simulink model "add_sine_waves"  (R2021b)
settings: Solver=VariableStepAuto  StartTime=0.0  StopTime=10.0  RelTol=1e-3
settings Model: Creator=emre-  LastModifiedBy=emre-

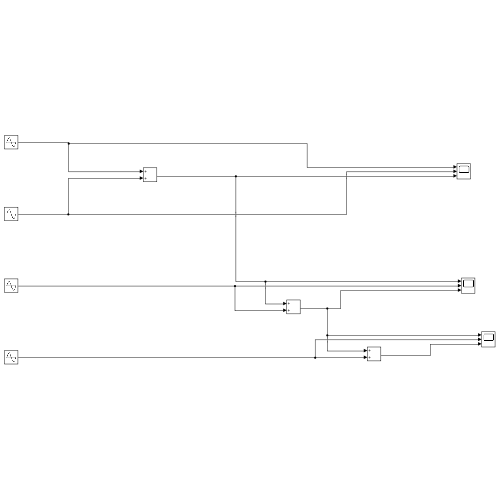
[thumbnail: Simulink's stored preview of the top-level diagram]
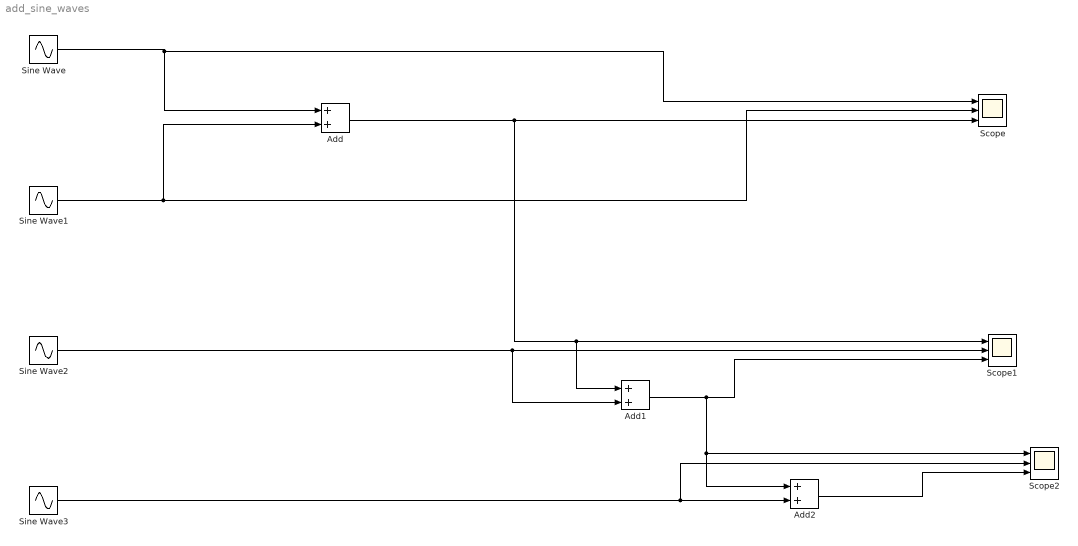
== system add_sine_waves ==
  Add : Sum
  Add1 : Sum
  Add2 : Sum
  Scope : Scope  NumInputPorts=3
  Scope1 : Scope  NumInputPorts=3
  Scope2 : Scope  NumInputPorts=3
  Sine Wave : Sin  SampleTime=0
  Sine Wave1 : Sin  Amplitude=1/3  Frequency=3  SampleTime=0
  Sine Wave2 : Sin  Amplitude=1/5  Frequency=5  SampleTime=0
  Sine Wave3 : Sin  Amplitude=1/7  Frequency=7  SampleTime=0
  wires:
  Sine Wave/1 -> Scope/1, Add/1
  Sine Wave1/1 -> Scope/2, Add/2
  Add/1 -> Scope1/1, Add1/1, Scope/3
  Sine Wave2/1 -> Scope1/2, Add1/2
  Add1/1 -> Scope2/1, Add2/1, Scope1/3
  Sine Wave3/1 -> Scope2/2, Add2/2
  Add2/1 -> Scope2/3
